simulink model "code_gen"  (Simulink 7.5)
settings: Solver=FixedStepDiscrete  StartTime=0.0  StopTime=10.0  FixedStep=0.001  RelTol=1e-3
InitFcn:
  | boat_constants
values from neighbouring files (symbols this model uses):
  InitialPoint = 0    [boat_constants.m]    (also in l2plus.m)
  IPStar = 0    [boat_constants.m]    (also in l2plus.m)
  ISA_g = 9.815    [boat_constants.m]
  MaxDwnPthStar = 1    [boat_constants.m]    (also in l2plus.m)
  OC2max = 49999    [boat_constants.m]    (also in simulation_constants.m)
  switchDistance = 4    [boat_constants.m]    (also in l2plus.m)
  T_step = 0.01    [boat_constants.m]    (also in common.m)
  tanIntercept = tan( 45*pi/180 )    [boat_constants.m]    (also in l2plus.m)
  TStar = single(4.5)    [boat_constants.m]    (also in l2plus.m = single(2))
  Turn2Track = 0    [boat_constants.m]    (also in l2plus.m)
undefined symbols (not defined in the file or in its folder): buildAndCheckMessage, buildAndCheckSentence, DiscIntNeverNeededParam, ecan1_buffered_transmit_matlab, ecan1_init, getGpsMainData, getSensorData, u1, y1
libraries: simulink x49, dsPICdrivers x22, simulink_need_slupdate x6, microSimulink x4, aerolibconvert2 x3
(part 3 of 3)

== system code_gen/Propulsion Outputs/To Drive Motor/uint8 combiner1 ==
  high-order : Inport  OutDataType=sfix(16)  OutScaling=2^0
  low-order : Inport  Port=2  OutDataType=sfix(16)  OutScaling=2^0
  Bitwise Operator : simulink/Logic and Bit Operations/Bitwise Operator  logicop=OR  UseBitMask=off  NumInputPorts=2  BitMask=bin2dec('11011001')  BitMaskRealWorld=Stored Integer
  Data Type Conversion : DataTypeConversion  OutDataTypeMode=uint16  OutDataType=sfix(16)  OutScaling=2^0  OutDataTypeStr=uint16
  Data Type Conversion1 : DataTypeConversion  OutDataTypeMode=uint16  OutDataType=sfix(16)  OutScaling=2^0  OutDataTypeStr=uint16
  Shift Arithmetic : simulink/Logic and Bit Operations/Shift Arithmetic  SystemSampleTime=-1  nBitShiftRight=-8  nBinPtShiftRight=0
  combined : Outport  OutDataType=sfix(16)  OutScaling=2^0
  wires:
  low-order/1 -> Data Type Conversion/1
  Bitwise Operator/1 -> combined/1
  high-order/1 -> Data Type Conversion1/1
  Shift Arithmetic/1 -> Bitwise Operator/2
  Data Type Conversion/1 -> Shift Arithmetic/1
  Data Type Conversion1/1 -> Bitwise Operator/1

== system code_gen/Propulsion Outputs/To Drive Motor/uint8 combiner2 ==
  high-order : Inport  OutDataType=sfix(16)  OutScaling=2^0
  low-order : Inport  Port=2  OutDataType=sfix(16)  OutScaling=2^0
  Bitwise Operator : simulink/Logic and Bit Operations/Bitwise Operator  logicop=OR  UseBitMask=off  NumInputPorts=2  BitMask=bin2dec('11011001')  BitMaskRealWorld=Stored Integer
  Data Type Conversion : DataTypeConversion  OutDataTypeMode=uint16  OutDataType=sfix(16)  OutScaling=2^0  OutDataTypeStr=uint16
  Data Type Conversion1 : DataTypeConversion  OutDataTypeMode=uint16  OutDataType=sfix(16)  OutScaling=2^0  OutDataTypeStr=uint16
  Shift Arithmetic : simulink/Logic and Bit Operations/Shift Arithmetic  SystemSampleTime=-1  nBitShiftRight=-8  nBinPtShiftRight=0
  combined : Outport  OutDataType=sfix(16)  OutScaling=2^0
  wires:
  Data Type Conversion1/1 -> Bitwise Operator/1
  Data Type Conversion/1 -> Shift Arithmetic/1
  Shift Arithmetic/1 -> Bitwise Operator/2
  high-order/1 -> Data Type Conversion1/1
  Bitwise Operator/1 -> combined/1
  low-order/1 -> Data Type Conversion/1

== system code_gen/Throttle Command/Mux Everything/Generate speed command ==
  In1 : Inport
  Bias1 : Bias  Bias=-7215
  Build speed command : Subsystem
  Data Type Conversion : DataTypeConversion  OutDataTypeMode=int32  OutDataType=sfix(16)  OutScaling=2^0  OutDataTypeStr=int32  ConvertRealWorld=Stored Integer (SI)
  Data Type Conversion1 : DataTypeConversion  OutDataTypeMode=int16  OutDataType=sfix(16)  OutScaling=2^0  OutDataTypeStr=int16
  Saturation1 : Saturate  UpperLimit=1023  LowerLimit=-1023
  Shift Arithmetic : simulink/Logic and Bit Operations/Shift Arithmetic  SystemSampleTime=-1  nBitShiftRight=1  nBinPtShiftRight=0
  Weighted Moving Average1 : simulink_need_slupdate/Weighted Moving Average  mgainval=[.5 .5]  vinit=0.0  samptime=-1  OutDataTypeStr=Inherit: Inherit via back propagation  OutDataType=sfix(16)  OutScaling=2^-10  DoSatur=off  GainDataType=uint(16)  MatRadixGroup=Best Precision: Matrix-wise  GainScaling=2^-10
  Out1 : Outport
  wires:
  Bias1/1 -> Shift Arithmetic/1
  Data Type Conversion/1 -> Bias1/1
  Shift Arithmetic/1 -> Data Type Conversion1/1
  Saturation1/1 -> Weighted Moving Average1/1
  Data Type Conversion1/1 -> Saturation1/1
  Weighted Moving Average1/1 -> Build speed command/1(CC)
  Build speed command/1(msg) -> Out1/1
  In1/1 -> Data Type Conversion/1

== system code_gen/Throttle Command/Trigger Events/Detect to/from zero ==
  hightime : Inport  OutDataType=sfix(16)  OutScaling=2^0
  Compare To Zero2 : simulink/Logic and Bit Operations/Compare To Zero  SystemSampleTime=-1  relop=>  LogicOutDataTypeMode=boolean  ZeroCross=off
  Compare To Zero3 : simulink/Logic and Bit Operations/Compare To Zero  SystemSampleTime=-1  relop===  LogicOutDataTypeMode=boolean  ZeroCross=off
  Compare To Zero4 : simulink/Logic and Bit Operations/Compare To Zero  SystemSampleTime=-1  relop=>  LogicOutDataTypeMode=boolean  ZeroCross=off
  Compare To Zero5 : simulink/Logic and Bit Operations/Compare To Zero  SystemSampleTime=-1  relop===  LogicOutDataTypeMode=boolean  ZeroCross=off
  Integer Delay : simulink/Discrete/Integer Delay  vinit=0.0  samptime=-1  NumDelays=1
  Logical Operator7 : Logic  AllPortsSameDT=off  OutDataTypeMode=boolean  OutDataTypeStr=boolean
  Logical Operator8 : Logic  AllPortsSameDT=off  OutDataTypeMode=boolean  OutDataTypeStr=boolean
  Went low : Outport  OutDataType=sfix(16)  OutScaling=2^0
  Went high : Outport  Port=2  OutDataType=sfix(16)  OutScaling=2^0
  wires:
  Logical Operator7/1 -> Went low/1
  Compare To Zero4/1 -> Logical Operator8/2
  Compare To Zero5/1 -> Logical Operator8/1
  Compare To Zero3/1 -> Logical Operator7/2
  Compare To Zero2/1 -> Logical Operator7/1
  Integer Delay/1 -> Compare To Zero2/1, Compare To Zero5/1
  hightime/1 -> Integer Delay/1, Compare To Zero3/1, Compare To Zero4/1
  Logical Operator8/1 -> Went high/1

== system code_gen/Autonomous Controller/Throttle Command/Mux Everything/Generate speed command ==
  In1 : Inport
  Bias1 : Bias  Bias=-7215
  Build speed command : Subsystem
  Data Type Conversion : DataTypeConversion  OutDataTypeMode=int32  OutDataType=sfix(16)  OutScaling=2^0  OutDataTypeStr=int32  ConvertRealWorld=Stored Integer (SI)
  Data Type Conversion1 : DataTypeConversion  OutDataTypeMode=int16  OutDataType=sfix(16)  OutScaling=2^0  OutDataTypeStr=int16
  Saturation1 : Saturate  UpperLimit=1023  LowerLimit=-1023
  Shift Arithmetic : simulink/Logic and Bit Operations/Shift Arithmetic  SystemSampleTime=-1  nBitShiftRight=1  nBinPtShiftRight=0
  Weighted Moving Average1 : simulink_need_slupdate/Weighted Moving Average  mgainval=[.5 .5]  vinit=0.0  samptime=-1  OutDataTypeStr=Inherit: Inherit via back propagation  OutDataType=sfix(16)  OutScaling=2^-10  DoSatur=off  GainDataType=uint(16)  MatRadixGroup=Best Precision: Matrix-wise  GainScaling=2^-10
  Out1 : Outport
  wires:
  In1/1 -> Data Type Conversion/1
  Build speed command/1(msg) -> Out1/1
  Weighted Moving Average1/1 -> Build speed command/1(CC)
  Data Type Conversion1/1 -> Saturation1/1
  Saturation1/1 -> Weighted Moving Average1/1
  Shift Arithmetic/1 -> Data Type Conversion1/1
  Data Type Conversion/1 -> Bias1/1
  Bias1/1 -> Shift Arithmetic/1

== system code_gen/Autonomous Controller/Throttle Command/Trigger Events/Detect to/from zero ==
  hightime : Inport  OutDataType=sfix(16)  OutScaling=2^0
  Compare To Zero2 : simulink/Logic and Bit Operations/Compare To Zero  SystemSampleTime=-1  relop=>  LogicOutDataTypeMode=boolean  ZeroCross=off
  Compare To Zero3 : simulink/Logic and Bit Operations/Compare To Zero  SystemSampleTime=-1  relop===  LogicOutDataTypeMode=boolean  ZeroCross=off
  Compare To Zero4 : simulink/Logic and Bit Operations/Compare To Zero  SystemSampleTime=-1  relop=>  LogicOutDataTypeMode=boolean  ZeroCross=off
  Compare To Zero5 : simulink/Logic and Bit Operations/Compare To Zero  SystemSampleTime=-1  relop===  LogicOutDataTypeMode=boolean  ZeroCross=off
  Integer Delay : simulink/Discrete/Integer Delay  vinit=0.0  samptime=-1  NumDelays=1
  Logical Operator7 : Logic  AllPortsSameDT=off  OutDataTypeMode=boolean  OutDataTypeStr=boolean
  Logical Operator8 : Logic  AllPortsSameDT=off  OutDataTypeMode=boolean  OutDataTypeStr=boolean
  Went low : Outport  OutDataType=sfix(16)  OutScaling=2^0
  Went high : Outport  Port=2  OutDataType=sfix(16)  OutScaling=2^0
  wires:
  Logical Operator8/1 -> Went high/1
  hightime/1 -> Compare To Zero4/1, Compare To Zero3/1, Integer Delay/1
  Integer Delay/1 -> Compare To Zero5/1, Compare To Zero2/1
  Compare To Zero2/1 -> Logical Operator7/1
  Compare To Zero3/1 -> Logical Operator7/2
  Compare To Zero5/1 -> Logical Operator8/1
  Compare To Zero4/1 -> Logical Operator8/2
  Logical Operator7/1 -> Went low/1

== system code_gen/Throttle Command/Mux Everything/Generate speed command/Build speed command ==
  CC : Inport  OutDataType=sfix(16)  OutScaling=2^0
  Constant : Constant  OutDataTypeMode=int8  OutDataType=sfix(16)  OutScaling=2^0  OutDataTypeStr=int8
  Constant1 : Constant  Value=0  OutDataTypeMode=int8  OutDataType=sfix(16)  OutScaling=2^0  OutDataTypeStr=int8
  Constant2 : Constant  Value=0  OutDataTypeMode=int8  OutDataType=sfix(16)  OutScaling=2^0  OutDataTypeStr=int8
  Constant3 : Constant  Value=5  OutDataTypeMode=int8  OutDataType=sfix(16)  OutScaling=2^0  OutDataTypeStr=int8
  Data Type Conversion : DataTypeConversion  OutDataTypeMode=uint8  OutDataType=sfix(16)  OutScaling=2^0  OutDataTypeStr=uint8  ConvertRealWorld=Stored Integer (SI)
  Extract Bits : simulink/Logic and Bit Operations/Extract Bits  SystemSampleTime=-1  bitsToExtract=Upper half  numBits=8  bitIdxRange=[24 31]  outScalingMode=Treat bit field as an integer
  Extract Bits1 : simulink/Logic and Bit Operations/Extract Bits  SystemSampleTime=-1  bitsToExtract=Lower half  numBits=8  bitIdxRange=[16 23]  outScalingMode=Treat bit field as an integer
  myMux : Stateflow chart  TreatAsAtomicUnit=on
  msg : Outport  OutDataType=sfix(16)  OutScaling=2^0
  wires:
  CC/1 -> Extract Bits/1, Extract Bits1/1
  Data Type Conversion/1 -> msg/1
  Constant2/1 -> myMux/6(u6)
  Constant1/1 -> myMux/5(u5)
  myMux/1(y) -> Data Type Conversion/1
  Extract Bits1/1 -> myMux/4(u4)
  Extract Bits/1 -> myMux/3(u3)
  Constant3/1 -> myMux/2(u2)
  Constant/1 -> myMux/1(u1)

== system code_gen/Autonomous Controller/Throttle Command/Mux Everything/Generate speed command/Build speed command ==
  CC : Inport  OutDataType=sfix(16)  OutScaling=2^0
  Constant : Constant  OutDataTypeMode=int8  OutDataType=sfix(16)  OutScaling=2^0  OutDataTypeStr=int8
  Constant1 : Constant  Value=0  OutDataTypeMode=int8  OutDataType=sfix(16)  OutScaling=2^0  OutDataTypeStr=int8
  Constant2 : Constant  Value=0  OutDataTypeMode=int8  OutDataType=sfix(16)  OutScaling=2^0  OutDataTypeStr=int8
  Constant3 : Constant  Value=5  OutDataTypeMode=int8  OutDataType=sfix(16)  OutScaling=2^0  OutDataTypeStr=int8
  Data Type Conversion : DataTypeConversion  OutDataTypeMode=uint8  OutDataType=sfix(16)  OutScaling=2^0  OutDataTypeStr=uint8  ConvertRealWorld=Stored Integer (SI)
  Extract Bits : simulink/Logic and Bit Operations/Extract Bits  SystemSampleTime=-1  bitsToExtract=Upper half  numBits=8  bitIdxRange=[24 31]  outScalingMode=Treat bit field as an integer
  Extract Bits1 : simulink/Logic and Bit Operations/Extract Bits  SystemSampleTime=-1  bitsToExtract=Lower half  numBits=8  bitIdxRange=[16 23]  outScalingMode=Treat bit field as an integer
  myMux : Stateflow chart  TreatAsAtomicUnit=on
  msg : Outport  OutDataType=sfix(16)  OutScaling=2^0
  wires:
  Constant/1 -> myMux/1(u1)
  Constant3/1 -> myMux/2(u2)
  Extract Bits/1 -> myMux/3(u3)
  Extract Bits1/1 -> myMux/4(u4)
  myMux/1(y) -> Data Type Conversion/1
  Constant1/1 -> myMux/5(u5)
  Constant2/1 -> myMux/6(u6)
  Data Type Conversion/1 -> msg/1
  CC/1 -> Extract Bits1/1, Extract Bits/1

== matlab function Autonomous Controller/Rudder Command/Embedded MATLAB Function1 ==
  data: lat_accel input double; rudder output single; wheelbase parameter double; velocity input double size=3
function rudder = fcn(lat_accel, wheelbase, velocity)
%#eml
% the -99/99 lat_accel checks for maximum possible accel. This should correspond to maximum rudder deflection.

rudder = single(0);

if (norm(velocity) == 0 || lat_accel == 0)
    rudder = single(0);
elseif (lat_accel == 99) 
    rudder = single(pi/2);
elseif (lat_accel == -99) 
    rudder = single(-pi/2);
else
    rudder = atan(lat_accel*wheelbase/norm(velocity)^2);
end

== matlab function Autonomous Controller/Throttle Command/Mux Everything/Generate speed command/Build speed command/myMux ==
  data: u1 input double; y output double; u2 input double; u3 input double; u4 input double; u5 input double; u6 input double
function y = myMux(u1, u2, u3, u4, u5, u6)
y = [u1(1); u2(1); u3(1); u4(1); u5(1); u6(1);];

== matlab function Autonomous Controller/Rudder Command/Waypoint Controller ==
  data: waypoint_0 output single size=3; waypoint_1 output single size=3; waypoints parameter single; switchTrigger input boolean; mode input uint8
function [waypoint_0, waypoint_1] = fcn(waypoints, switchTrigger, mode)
%#eml

persistent index_0 index_1; % Store the indices for waypoints 0 & 1 respectively
persistent direction; % Keep track of the direction for patrol mode

% Make sure we have at least two waypoints to output
assert(size(waypoints,1) >= 2);

% Inititalize to the first waypoint
if isempty(index_0)
    index_0 = 1;
end
if isempty(index_1)
    index_1 = 2;
end
if isempty(direction)
    direction = 1;
end
 
% Increment our waypoint index if we're told to.
if switchTrigger
    switch mode
        case 0 % Halt mode
            if size(waypoints,1) >= index_1 + 1
                index_0 = index_1;
                index_1 = index_1 + 1;
            end
        case 1 % Loop mode
            % We either continue moving forward through the waypoints...
            if size(waypoints,1) >= index_1 + 1
                index_0 = index_1;
                index_1 = index_1 + 1;
            % Or we wrap-around to the starting waypoint
            else
                index_0 = index_1;
                index_1 = 1;
            end
        case 2 % Patrol mode
            if direction == 1 % For the forwards direction
                % We either continue moving forwards through the waypoints...
                if size(waypoints,1) >= index_1 + 1
                    index_0 = index_1;
                    index_1 = index_1 + 1;
                % Or we start to go backwards
                else
                    index_0 = index_1;
                    index_1 = index_1 - 1;
                    direction = 0;
                end
            elseif direction == 0 % For the reverse direction
                % We either continue moving backwards through the waypoints...
                if index_1 - 1 >= 1
                    index_0 = index_1;
                    index_1 = index_1 - 1;
                % Or we start to go forwards
                else
                    index_0 = index_1;
                    index_1 = index_1 + 1;
                    direction = 1;
                end
            end
    end
end

waypoint_0 = waypoints(index_0,:)';
waypoint_1 = waypoints(index_1,:)';

== matlab function Autonomous Controller/Throttle Command/Mux Everything/Select data packet ==
  data: y output double; dis input double; en input double
function y = fcn(dis, en)
% This block controls the switch selecting between enable, 
% disable, and speed commands. If disable and enable are
% both set high, disable overrides anything else.

y = uint8(3);
if dis == 1
    y = uint8(1);
elseif en == 1
    y = uint8(2);
end

== matlab function Throttle Command/Mux Everything/Generate speed command/Build speed command/myMux ==
  data: u1 input double; y output double; u2 input double; u3 input double; u4 input double; u5 input double; u6 input double
function y = myMux(u1, u2, u3, u4, u5, u6)
y = [u1(1); u2(1); u3(1); u4(1); u5(1); u6(1);];

== matlab function GPS/Embedded MATLAB Function ==
  data: u input double; a output double; b output double; c output double
function [a,b,c] = fcn(u)
%#eml
a = uint8(bitshift(bitand(uint32(u),61440),-12));
b = uint8(bitshift(bitand(uint32(u),3840),-8));
c = uint8(bitshift(bitand(uint32(u),240),-4));

== matlab function Autonomous Controller/Rudder Command/L2 Plus ref WP1 ==
  data: triggerSwitch output boolean; WP0 input single; WP1 input single; Puav input single size=3; Vxyz input single size=3; switchDistance parameter double size=1; ISA_g parameter double; tanIntercept parameter double; MaxDwnPthStar parameter double; Turn2Track parameter double; InitialPoint parameter double; IPStar parameter double; TStar parameter double; as_c output single; L2Vec output single
function [triggerSwitch, as_c, L2Vec] = L2PlusWP1(WP0, WP1, Puav, Vxyz, switchDistance, ...
    ISA_g, tanIntercept, MaxDwnPthStar,Turn2Track,...
    InitialPoint, IPStar, TStar)
%==============================
%     computes bank angle command for following a straight line
%     by creating an aim point that may be more than L2 away 
%     from the UAV. The aim point is (usually) farther along the path 
%     toward WP1 than the UAV, and the intercept
%     angle is less than or equal to a specified value. This limits the intercept
%     angle even when the UAV is within L2 of the path.
%     See L2PlusWP1.m for details
    
%         INPUTS   
%             T1      unit vector WP0-->WP1
%             N1      normal to T1
%             WP0     position of "from" waypoint. only needed to set an InitialPoint
%             WP1     position of WP1, active waypoint
%             Puav    position of UAV
%             Vxyz    Inertial velocity
%             switchDistance distance from WP1 to switch to WP2

%         PARAMETERS
%             ISA_g   gravity
%             tanIntercept  tangent of intercept angle
%             MaxDwnPthStar L2 multiplier to determmine downpath aimpoint
%             Turn2Track    true to turn toward T1 instead of L2
%             InitialPoint  true if no line tracking at first--fly direct to some initial point
%             IPStar        L2 multiplier to determing distance of IP from first WP0
%             Tstar         was called L2Base, time constant of response
%             
%         OUTPUTS
%             phi_c   commanded bank angle (positive is a starboard turn)
%             L2Vec   L2 vector toward aim point
%             as_c    commanded lateral acceleration
%             Groundspeed 
%             IP1     position of IP for plotting purposes. IP1(3) = -999 if no IP exists

    persistent IPActive;  %true if flying toward IP
    persistent IP; % location of initial point
%     if (~SwitchMode)
%         phi_c = single(0);
%         L2Vec = single(zeros(3,1));
%         as_c = single(0);
%         Groundspeed = sqrt(Vxyz(1)*Vxyz(1) + Vxyz(2)*Vxyz(2));
%         IPActive = IPActive;
%     end
%     
    triggerSwitch = false;
    Pwp1 = single(zeros(3,1));
    Pe_y = single(0);
    Dist2WP1 = single(0);
    MinDownPath = single(0);
    Dist2WPSwitch = single(0);
    L2DownPath = single(0);
    L2ToT = single(zeros(3,1));
    L2Vec = single(zeros(3,1));
    IP1 = single([0; 0;-999]); %signal for no IP
    
    Pne = [Puav(1); Puav(2); 0]; %horizontal position
    Vne = [Vxyz(1); Vxyz(2); 0]; % horizontal velocity
    Groundspeed = norm(Vne);
    L2 = single(TStar*Groundspeed);
    WP0ne = single(zeros(3,1));
    
% Calculate N1 and T1
assert(norm(WP1 - WP0) ~= 0);
T1 = WP1-WP0;
T1 = T1/norm(T1);
N1 = [-T1(2); T1(1); 0];
    
%     initialize IP
    if (isempty(IPActive))
        if (InitialPoint)
%             IP is set relative to the first "from" waypoint
            IPActive = -1;
            IP = [WP0(1); WP0(2); 0] - L2*IPStar*T1;
            
            if (norm(IP-Pne) < .001)
                IPActive = 0;
                IP = single([0; 0; -999]);
            end
        else
            IPActive = 0;
            IP = single([0; 0;-999]); %signal for no IP
        end
    end
    IP1 = IP;
    
    
    if (IPActive)
%         no line tracking, direct to IP
        L2Vec = L2*(IP - Pne)/norm(IP - Pne);
%         check to see if at the IP to terminate this mode
        if norm(IP - Pne) < .1*L2
            IPActive = 0;
        end
    else
         if (Pne(1) < 2)
             IP1 = IP1;
         end
%         IP not active, track WP lines
        WPOne = [WP1(1); WP1(2); 0];
        Pwp1 = Pne - [WP1(1); WP1(2); 0]; % position of UAV relative to WP1
        Pe_y = single(Pwp1'*N1); % cross track error
        Dist2WP1 = -single(Pwp1'*T1); % distance to WP1

%         minimum down path distance for Aim Point intersection on T
%         is determined by the intercept angle but limited 
%         in case of very distant intecepts to MaxDwnPthStar*L2
        MinDownPath = single ( min( abs(Pe_y)/tanIntercept, MaxDwnPthStar*L2)); 
        Dist2WPSwitch = Dist2WP1 - switchDistance;
        if ( abs(Pe_y) > L2 )
    %             Make sure aimpoint is no closer to waypoint than calculated switch point.
            L2DownPath = MinDownPath;
        else
    %             within L2 of T and Dist2WPSwitch >= 0, but limit angle of L2 wrt T
            L2DownPath = (max(MinDownPath, (sqrt( L2^2 - Pe_y^2 ))));
        end
        
        if ( Dist2WPSwitch < 0 )
            triggerSwitch = true;
        end
        
         % vector from Pwp1 to aim point on T1
         L2ToT = single(( Dist2WP1 - L2DownPath )*(-T1) - Pwp1);
         if (norm(L2ToT) < .001)
             L2Vec = L2*T1;
         else
            L2Vec = single(L2*( L2ToT/norm(L2ToT) )); % limit size to L2
         end
    %         L2Vec = L2ToT;
%         dummy statements
    end
    Zprod = single(Vxyz(1)*L2Vec(2) - Vxyz(2)*L2Vec(1)); %Z component of cross product
    sinEta = single(Zprod/(Groundspeed*L2));

    as_c = single(2*Groundspeed^2/(L2)*sinEta);
%         bank angle limits outside of this block
    phi_c = single(atan(as_c/ISA_g));

%         now override bank angle if heading in the wrong direction
    if ( Turn2Track && Dist2WPSwitch > 0 && ~IPActive ) 
%             turn to track not L2, gives min displacement from track
        if ( T1'*Vxyz < 0 )
            if ( Pe_y > 0 )
                phi_c = single(+pi/2);
                as_c = single(99);
            else
                phi_c = single(-pi/2);
                as_c = single(-99);
            end
        end
     else
%           turn toward L2, give min displacement toward WP0
        if ( L2Vec'*Vxyz < 0 )
            if ( sinEta < 0 )
                phi_c = single(-pi/2); 
                as_c = single(-99);
            else
                phi_c = single(+pi/2);
                as_c = single(99);
            end
        end
    end
end

== matlab function Propulsion Outputs/To Drive Motor/myMux ==
  data: u1 input double; y output double; u2 input double; u3 input double; u4 input double; u5 input double
function y = myMux(u1, u2, u3, u4, u5)
u5_u16 = uint16(u5);
y = uint16([u1(1); u2(1); u3(1); u4(1); 0; 0; 0; 0;]);

len = length(u5);
if len > 1
    y(5) = bitor(bitshift(u5_u16(1),8),u5_u16(2));
elseif len > 0
    y(5) = u5_u16(1);
end
if len > 3
    y(6) = bitor(bitshift(u5_u16(3),8),u5_u16(4));
elseif len > 2
    y(6) = u5_u16(3);
end
if len > 5
    y(7) = bitor(bitshift(u5_u16(5),8),u5_u16(6));
elseif len > 4
    y(7) = u5_u16(5);
end
if len > 7
    y(8) = bitor(bitshift(u5_u16(7),8),u5_u16(8));
elseif len > 6
    y(8) = u5_u16(7);
end

== matlab function GPS/Embedded MATLAB Function1 ==
  data: u input double; a output double; b output double; c output double
function [a,b,c] = fcn(u)
%#eml
a = uint8(bitshift(bitand(uint32(u),61440),-12));
b = uint8(bitshift(bitand(uint32(u),3840),-8));
c = uint8(bitshift(bitand(uint32(u),240),-4));

== matlab function Throttle Command/Mux Everything/Select data packet ==
  data: y output double; dis input double; en input double
function y = fcn(dis, en)
% This block controls the switch selecting between enable, 
% disable, and speed commands. If disable and enable are
% both set high, disable overrides anything else.

y = uint8(3);
if dis == 1
    y = uint8(1);
elseif en == 1
    y = uint8(2);
end
